simulink model "laba_4"  (Simulink 9.2)
settings: Solver=FixedStepAuto  StartTime=0.0  StopTime=130  FixedStep=0.0001  RelTol=1e-3  EnableMultiTasking=on
settings Model: Creator=student  LastModifiedBy=murad  SnapshotInterval=100
settings OptimizationCC: ExpressionDepthLimit=2147483647
settings DebuggingCC: SolverPrmCheckMsg=warning

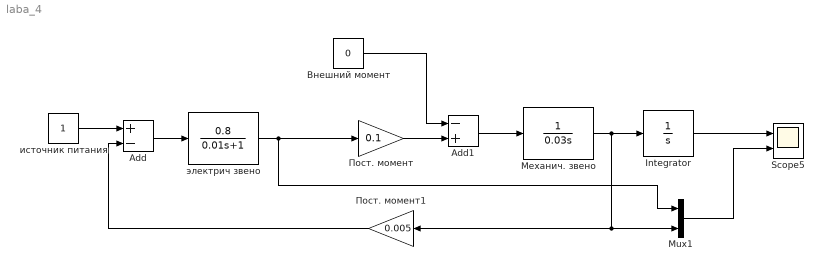
== system laba_4 ==
  Add : Sum  Inputs=+-
  Add1 : Sum  Inputs=-+
  Integrator : Integrator
  Mux1 : Mux  Inputs=2
  Scope5 : Scope  NumInputPorts=2
  Внешний момент : Constant  Value=0
  Механич. звено : TransferFcn  Denominator=[0.03 0]
  Пост. момент : Gain  Gain=0.1
  Пост. момент1 : Gain  Gain=0.005
  источник питания : Constant
  электрич звено : TransferFcn  Numerator=[0.8]  Denominator=[0.01 1]
  wires:
  источник питания/1 -> Add/1
  Add/1 -> электрич звено/1
  электрич звено/1 -> Mux1/1, Пост. момент/1
  Пост. момент/1 -> Add1/2
  Внешний момент/1 -> Add1/1
  Add1/1 -> Механич. звено/1
  Механич. звено/1 -> Mux1/2, Пост. момент1/1, Integrator/1
  Пост. момент1/1 -> Add/2
  Mux1/1 -> Scope5/2
  Integrator/1 -> Scope5/1
